simulink model "DataCenterSim"  (R2024b)
settings: Solver=VariableStepAuto  StartTime=0.0  StopTime=SimTime  MaxStep=MaxStep  RelTol=RelTol
values from neighbouring files (symbols this model uses):
  alpha = 1    [DataCenter.m]
  K = K_base    [DataCenter.m]
  Pref = 0.5*mean(PLstep_raw)    [DataCenter.m]
  Px = 2*max(PLstep_raw)    [DataCenter.m]
settings Model: Creator=elino  LastModifiedBy=Elinor
settings DataIOCC: SaveOutput=off  SignalLogging=off  DSMLogging=off  SaveTime=off  ReturnWorkspaceOutputs=off

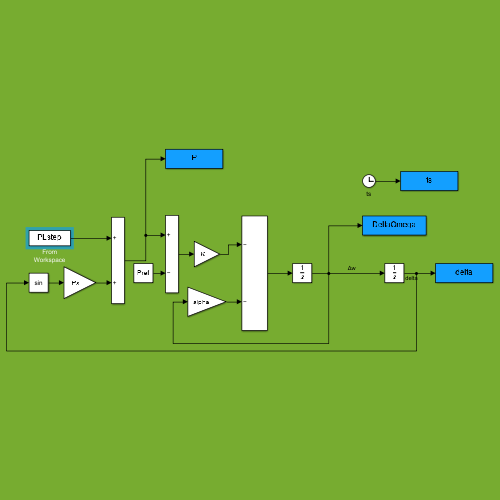
[thumbnail: Simulink's stored preview of the top-level diagram]
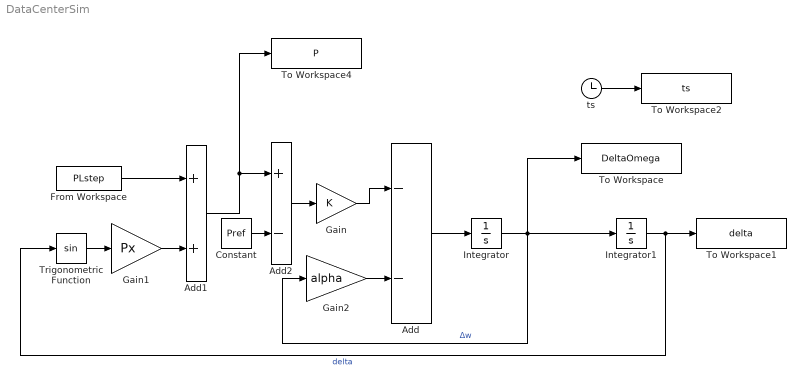
== system DataCenterSim ==
  Add : Sum  Inputs=--
  Add1 : Sum
  Add2 : Sum  Inputs=+-
  Constant : Constant  Value=Pref
  From Workspace : FromWorkspace  VariableName=PLstep
  Gain : Gain  Gain=K
  Gain1 : Gain  Gain=Px
  Gain2 : Gain  Gain=alpha
  Integrator : Integrator
  Integrator1 : Integrator  InitialCondition=asin(Pref/Px)
  To Workspace : ToWorkspace  VariableName=DeltaOmega  SampleTime=-1
  To Workspace1 : ToWorkspace  VariableName=delta  SampleTime=-1
  To Workspace2 : ToWorkspace  VariableName=ts  SampleTime=-1
  To Workspace4 : ToWorkspace  VariableName=P  SampleTime=-1
  Trigonometric Function : Trigonometry
  ts : Clock
  wires:
  Integrator/1 -> Integrator1/1, To Workspace/1, Gain2/1  "Δw"
  Integrator1/1 -> To Workspace1/1, Trigonometric Function/1  "delta"
  Gain/1 -> Add/1
  Add/1 -> Integrator/1
  Trigonometric Function/1 -> Gain1/1
  ts/1 -> To Workspace2/1
  Gain2/1 -> Add/2
  Constant/1 -> Add2/2
  Gain1/1 -> Add1/2
  Add1/1 -> To Workspace4/1, Add2/1
  Add2/1 -> Gain/1
  From Workspace/1 -> Add1/1
